simulink model "TASK1_rotating"  (R2022b)
settings: Solver=VariableStepAuto  StartTime=0.0  StopTime=3  RelTol=1e-3
values from neighbouring files (symbols this model uses):
  m = 12    [MPC_Controller.m]    (also in QP_Controller.m; TASK1_rotating_mpc.m; TASK1_walking_backward_mpc.m; TASK1_walking_forward_mpc.m)
  N = 10    [MPC_Controller.m]
undefined symbols (not defined in the file or in its folder): TASK1_rotating_mpc, X, Y, Z
libraries: sm_lib x188, nesl_utility x122, simulink x1
(part 1 of 6)
settings Model: Creator=gabemaymon  LastModifiedBy=brendanmorrison
settings ModelReferenceCC: EnableRefExpFcnMdlSchedulingChecks=on

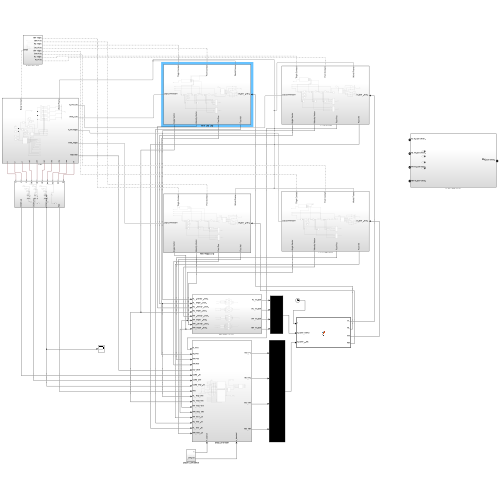
[thumbnail: Simulink's stored preview of the top-level diagram]
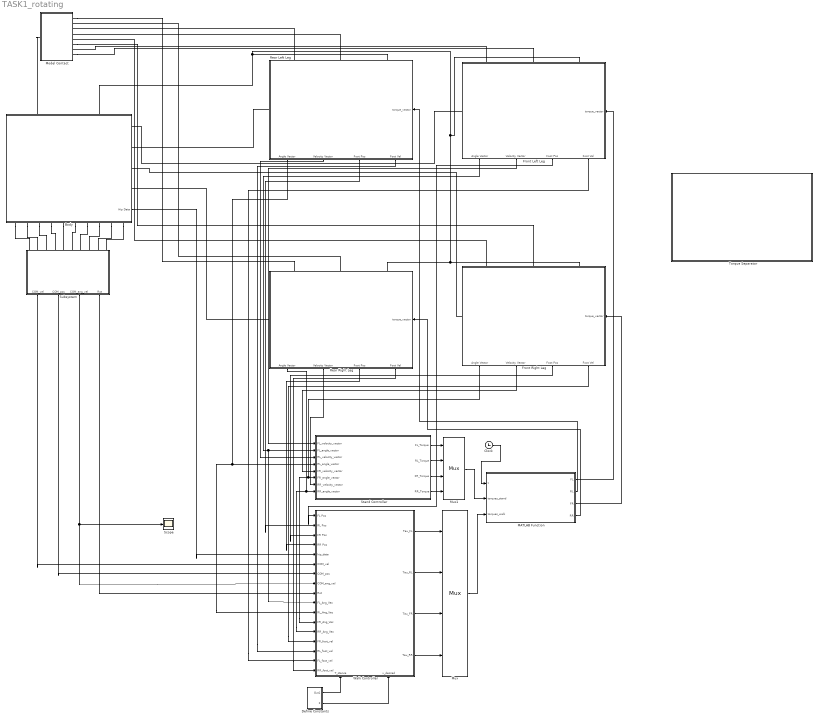
== system TASK1_rotating ==
  Body : Subsystem
      settings: PortSchema="{\"entries\":[{\"content\":{\"sides\":[{\"content\":{\"connectorIds\":[]},\"type\":\"ConnectorPlacement.EquallySpacedRectSide\",\"uuid\":\"3a53cbab-bcad-44fb-8467-9fb9b9a86323\"},{\"content\":{\"connectorIds\":[\"RConn1\",\"RConn2\",\"RConn3\",\"RConn4\",\"Out1\"],\"side\":\"RIGHT\"},\"type\":\"ConnectorPlacement.EquallySpacedRectSide\",\"uuid\":\"37b4c9a2-a58b-45a3-99d3-aa4f692e4db6\"},{\"content\":{\"connectorIds\":[\"LConn1\",\"LConn2\"],\"side\":\"TOP\"},\"type\":\"ConnectorPlacement.EquallySpacedRectSide\",\"uuid\":\"5dbc175b-de34-48ce-a2f5-f786354f8d9f\"},{\"content\":{\"connectorIds\":[\"RConn5\",\"RConn6\",\"RConn7\",\"RConn8\",\"RConn9\",\"RConn10\",\"RConn11\",\"RConn12\",\"RConn13\",\"RConn14\"],\"side\":\"BOTTOM\"},\"type\":\"ConnectorPlacement.EquallySpacedRectSide\",\"uuid\":\"77deabef-97a2-4647-8aef-301d0256e7d8\"}]},\"type\":\"ConnectorPlacement.EquallySpacedConnector\",\"uuid\":\"c3f44b19-9cb7-4370-b97a-4164cc5cfb48\"}],\"packageUris\":[\"http://schema.mathworks.com/mf0/Connector/R2020b\"],\"version\":\"1.0\"}"
  Clock : Clock
  Define Constants : Subsystem
  Front Left Leg : Subsystem
      settings: PortSchema="{\"entries\":[{\"content\":{\"sides\":[{\"content\":{\"connectorIds\":[\"LConn1\"]},\"type\":\"ConnectorPlacement.EquallySpacedRectSide\",\"uuid\":\"58990e36-5185-4bfb-924f-3ea489e575b7\"},{\"content\":{\"connectorIds\":[\"In1\"],\"side\":\"RIGHT\"},\"type\":\"ConnectorPlacement.EquallySpacedRectSide\",\"uuid\":\"00c4eac4-622f-4601-a916-f460578a2921\"},{\"content\":{\"connectorIds\":[\"LConn2\",\"LConn3\",\"LConn4\"],\"side\":\"TOP\"},\"type\":\"ConnectorPlacement.EquallySpacedRectSide\",\"uuid\":\"312df89b-6b71-4241-907b-a86e47405529\"},{\"content\":{\"connectorIds\":[\"Out1\",\"Out2\",\"Out3\",\"Out4\"],\"side\":\"BOTTOM\"},\"type\":\"ConnectorPlacement.EquallySpacedRectSide\",\"uuid\":\"0aae8fe1-113f-457b-a27e-e9cd9e6560df\"}]},\"type\":\"ConnectorPlacement.EquallySpacedConnector\",\"uuid\":\"0675262f-03c2-4ace-8aed-4bc959055a73\"}],\"packageUris\":[\"http://schema.mathworks.com/mf0/Connector/R2020b\"],\"version\":\"1.0\"}"
  Front Right Leg : Subsystem
      settings: PortSchema="{\"entries\":[{\"content\":{\"sides\":[{\"content\":{\"connectorIds\":[\"LConn1\"]},\"type\":\"ConnectorPlacement.EquallySpacedRectSide\",\"uuid\":\"58990e36-5185-4bfb-924f-3ea489e575b7\"},{\"content\":{\"connectorIds\":[\"In1\"],\"side\":\"RIGHT\"},\"type\":\"ConnectorPlacement.EquallySpacedRectSide\",\"uuid\":\"00c4eac4-622f-4601-a916-f460578a2921\"},{\"content\":{\"connectorIds\":[\"LConn2\",\"LConn3\",\"LConn4\"],\"side\":\"TOP\"},\"type\":\"ConnectorPlacement.EquallySpacedRectSide\",\"uuid\":\"312df89b-6b71-4241-907b-a86e47405529\"},{\"content\":{\"connectorIds\":[\"Out1\",\"Out2\",\"Out3\",\"Out4\"],\"side\":\"BOTTOM\"},\"type\":\"ConnectorPlacement.EquallySpacedRectSide\",\"uuid\":\"d64aa42d-2533-4acc-8ebf-5037fee0448f\"}]},\"type\":\"ConnectorPlacement.EquallySpacedConnector\",\"uuid\":\"0675262f-03c2-4ace-8aed-4bc959055a73\"}],\"packageUris\":[\"http://schema.mathworks.com/mf0/Connector/R2020b\"],\"version\":\"1.0\"}"
  MATLAB Function : MATLAB Function  TreatAsAtomicUnit=on
  Model Contact : Subsystem
  Mux : Mux
  Mux1 : Mux
  Rear Left Leg : Subsystem
      settings: PortSchema="{\"entries\":[{\"content\":{\"sides\":[{\"content\":{\"connectorIds\":[\"LConn1\"]},\"type\":\"ConnectorPlacement.EquallySpacedRectSide\",\"uuid\":\"58990e36-5185-4bfb-924f-3ea489e575b7\"},{\"content\":{\"connectorIds\":[\"In1\"],\"side\":\"RIGHT\"},\"type\":\"ConnectorPlacement.EquallySpacedRectSide\",\"uuid\":\"00c4eac4-622f-4601-a916-f460578a2921\"},{\"content\":{\"connectorIds\":[\"LConn2\",\"LConn3\",\"LConn4\"],\"side\":\"TOP\"},\"type\":\"ConnectorPlacement.EquallySpacedRectSide\",\"uuid\":\"312df89b-6b71-4241-907b-a86e47405529\"},{\"content\":{\"connectorIds\":[\"Out1\",\"Out2\",\"Out3\",\"Out4\"],\"side\":\"BOTTOM\"},\"type\":\"ConnectorPlacement.EquallySpacedRectSide\",\"uuid\":\"ff870af0-d312-4050-99ba-9f73bd605133\"}]},\"type\":\"ConnectorPlacement.EquallySpacedConnector\",\"uuid\":\"0675262f-03c2-4ace-8aed-4bc959055a73\"}],\"packageUris\":[\"http://schema.mathworks.com/mf0/Connector/R2020b\"],\"version\":\"1.0\"}"
  Rear Right Leg : Subsystem
      settings: PortSchema="{\"entries\":[{\"content\":{\"sides\":[{\"content\":{\"connectorIds\":[\"LConn1\"]},\"type\":\"ConnectorPlacement.EquallySpacedRectSide\",\"uuid\":\"58990e36-5185-4bfb-924f-3ea489e575b7\"},{\"content\":{\"connectorIds\":[\"In1\"],\"side\":\"RIGHT\"},\"type\":\"ConnectorPlacement.EquallySpacedRectSide\",\"uuid\":\"00c4eac4-622f-4601-a916-f460578a2921\"},{\"content\":{\"connectorIds\":[\"LConn2\",\"LConn3\",\"LConn4\"],\"side\":\"TOP\"},\"type\":\"ConnectorPlacement.EquallySpacedRectSide\",\"uuid\":\"312df89b-6b71-4241-907b-a86e47405529\"},{\"content\":{\"connectorIds\":[\"Out1\",\"Out2\",\"Out3\",\"Out4\"],\"side\":\"BOTTOM\"},\"type\":\"ConnectorPlacement.EquallySpacedRectSide\",\"uuid\":\"f067581c-0bad-4e2f-b908-6a87aedcf8c1\"}]},\"type\":\"ConnectorPlacement.EquallySpacedConnector\",\"uuid\":\"0675262f-03c2-4ace-8aed-4bc959055a73\"}],\"packageUris\":[\"http://schema.mathworks.com/mf0/Connector/R2020b\"],\"version\":\"1.0\"}"
  Scope : Scope
  Stand Controller : Subsystem
  Subsystem : Subsystem
  Torque Separator : Subsystem
  Walk Controller : Subsystem
      settings: PortSchema="{\"entries\":[{\"content\":{\"sides\":[{\"content\":{\"connectorIds\":[\"In1\",\"In2\",\"In3\",\"In4\",\"In5\",\"In6\",\"In7\",\"In8\",\"In9\",\"In10\",\"In11\",\"In12\",\"In13\",\"In14\",\"In15\",\"In16\",\"In17\"]},\"type\":\"ConnectorPlacement.EquallySpacedRectSide\",\"uuid\":\"1e069285-b883-4306-9ce3-c9505cac6642\"},{\"content\":{\"connectorIds\":[\"Out1\",\"Out2\",\"Out3\",\"Out4\"],\"side\":\"RIGHT\"},\"type\":\"ConnectorPlacement.EquallySpacedRectSide\",\"uuid\":\"beeabf05-15da-47f0-a05e-e3bbb85a150c\"},{\"content\":{\"connectorIds\":[],\"side\":\"TOP\"},\"type\":\"ConnectorPlacement.EquallySpacedRectSide\",\"uuid\":\"4dc75ef0-3dc8-45e4-9a6b-759a39a8569b\"},{\"content\":{\"connectorIds\":[\"In18\",\"In19\"],\"side\":\"BOTTOM\"},\"type\":\"ConnectorPlacement.EquallySpacedRectSide\",\"uuid\":\"16e05f6d-d9c2-431a-98da-de6aa17a42c7\"}]},\"type\":\"ConnectorPlacement.EquallySpacedConnector\",\"uuid\":\"7eb70f55-b335-4fe2-939a-f221a9bcbcbb\"}],\"packageUris\":[\"http://schema.mathworks.com/mf0/Connector/R2020b\"],\"version\":\"1.0\"}"
  wires:
  Front Left Leg/2(Velocity Vector) -> Stand Controller/1(FL_velocity_vector)
  Front Left Leg/1(Angle Vector) -> Walk Controller/10(FL_Ang_Vec), Stand Controller/2(FL_angle_vector)
  Rear Left Leg/1(Angle Vector) -> Walk Controller/11(RL_Ang_Vec), Stand Controller/4(RL_angle_vector)
  Rear Left Leg/2(Velocity Vector) -> Stand Controller/3(RL_velocity_vector)
  Rear Right Leg/1(Angle Vector) -> Walk Controller/13(RR_Ang_Vec), Stand Controller/8(RR_angle_vector)
  Rear Right Leg/2(Velocity Vector) -> Stand Controller/7(RR_velocity_vector)
  Front Right Leg/1(Angle Vector) -> Walk Controller/12(FR_Ang_Vec), Stand Controller/6(FR_angle_vector)
  Front Right Leg/2(Velocity Vector) -> Stand Controller/5(FR_velocity_vector)
  Stand Controller/1(FL_Torque) -> Mux1/1
  Stand Controller/2(RL_Torque) -> Mux1/2
  Stand Controller/3(FR_Torque) -> Mux1/3
  Stand Controller/4(RR_Torque) -> Mux1/4
  Mux1/1 -> MATLAB Function/2(torques_stand)
  Mux/1 -> MATLAB Function/3(torques_walk)
  MATLAB Function/1(FL) -> Front Left Leg/1(torque_vector)
  MATLAB Function/3(FR) -> Front Right Leg/1(torque_vector)
  MATLAB Function/2(RL) -> Rear Left Leg/1(torque_vector)
  MATLAB Function/4(RR) -> Rear Right Leg/1(torque_vector)
  Front Left Leg/3(" Foot Pos") -> Walk Controller/1(FL Pos)
  Rear Left Leg/3(" Foot Pos") -> Walk Controller/2(RL Pos)
  Body/1(Hip Data) -> Walk Controller/5(hip_data)
  Subsystem/1(COM_vel) -> Walk Controller/6(COM_vel)
  Subsystem/2(COM_pos) -> Walk Controller/7(COM_pos)
  Subsystem/3(COM_ang_vel) -> Walk Controller/8(COM_ang_vel), Scope/1
  Subsystem/4(Rot) -> Walk Controller/9(Rot)
  Front Right Leg/3(" Foot Pos") -> Walk Controller/3(FR Pos)
  Rear Right Leg/3(" Foot Pos") -> Walk Controller/4(RR Pos)
  Define Constants/1(Out1) -> Walk Controller/18(T_stance)
  Define Constants/2(v_desired) -> Walk Controller/19(v_desired)
  Walk Controller/1(Tau_FL) -> Mux/1
  Walk Controller/2(Tau_RL) -> Mux/2
  Walk Controller/3(Tau_FR) -> Mux/3
  Walk Controller/4(Tau_RR) -> Mux/4
  Rear Left Leg/4(" Foot Vel") -> Walk Controller/15(RL_foot_vel)
  Rear Right Leg/4(" Foot Vel") -> Walk Controller/17(RR_foot_vel)
  Front Right Leg/4(" Foot Vel") -> Walk Controller/14(FR_foot_vel)
  Front Left Leg/4(" Foot Vel") -> Walk Controller/16(FL_foot_vel)
  Clock/1 -> MATLAB Function/1(t)
  connections:
  Model Contact/RConn1 -- Rear Right Leg/LConn2
  Rear Left Leg/LConn2 -- Model Contact/RConn3
  Front Right Leg/LConn2 -- Model Contact/RConn5
  Front Left Leg/LConn2 -- Model Contact/RConn7
  Rear Right Leg/LConn3 -- Model Contact/RConn2
  Rear Left Leg/LConn3 -- Model Contact/RConn4
  Model Contact/RConn6 -- Front Right Leg/LConn3
  Model Contact/RConn8 -- Front Left Leg/LConn3
  Model Contact/LConn1 -- Body/LConn1
  Front Right Leg/LConn1 -- Body/RConn3
  Rear Left Leg/LConn1 -- Body/RConn2
  Rear Right Leg/LConn1 -- Body/RConn4
  Front Left Leg/LConn1 -- Body/RConn1
  Body/LConn2 -- Front Left Leg/LConn4 -- Front Right Leg/LConn4 -- Rear Right Leg/LConn4 -- Rear Left Leg/LConn4
  Body/RConn5 -- Subsystem/LConn1
  Body/RConn6 -- Subsystem/LConn2
  Body/RConn7 -- Subsystem/LConn3
  Body/RConn8 -- Subsystem/LConn4
  Body/RConn9 -- Subsystem/LConn5
  Body/RConn10 -- Subsystem/LConn6
  Body/RConn11 -- Subsystem/LConn7
  Body/RConn12 -- Subsystem/LConn8
  Body/RConn13 -- Subsystem/LConn9
  Body/RConn14 -- Subsystem/LConn10

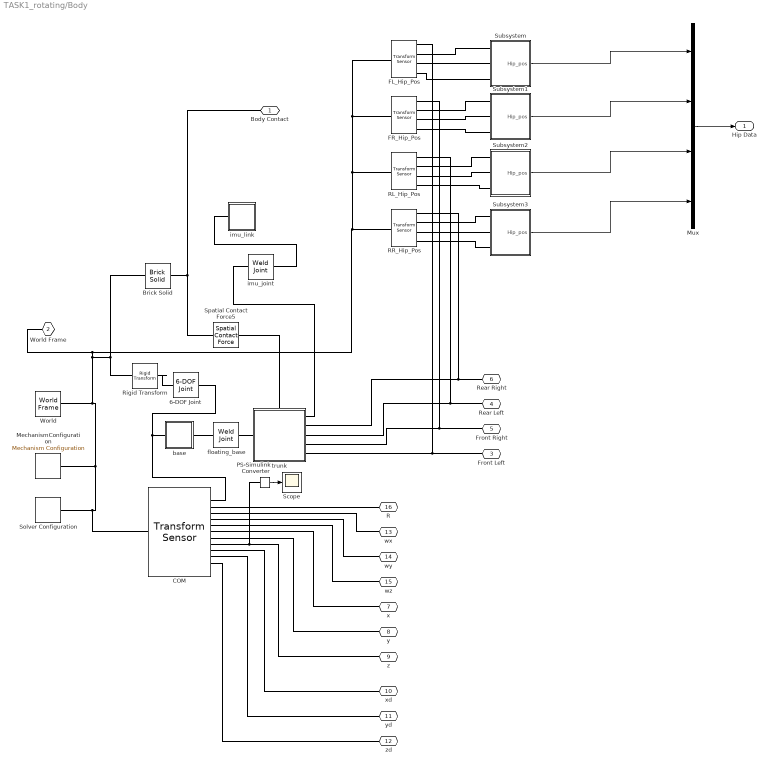
== system TASK1_rotating/Body ==
  " COM" : sm_lib/Frames and Transforms/Transform Sensor  MeasurementFrame=World  SenseAngle=off  SenseAxis=off  SenseQ=off  SenseR=on  SenseRotationSequence=off  RotationSequence=XYX  SenseOmegaX=on  SenseOmegaY=on  SenseOmegaZ=on  SenseQDot=off  SenseRDot=off  SenseAlphaX=off  SenseAlphaY=off  SenseAlphaZ=off  SenseQDDot=off  SenseRDDot=off  SenseX=on  SenseY=on  SenseZ=on  SenseRad=off  SenseAzim=off  SenseDist=off  SenseInc=off  SenseXDot=on  SenseYDot=on  SenseZDot=on  SenseRadDot=off  SenseAzimDot=off  SenseDistDot=off  SenseIncDot=off  SenseXDDot=off  SenseYDDot=off  SenseZDDot=off  SenseRadDDot=off  SenseAzimDDot=off  SenseDistDDot=off  SenseIncDDot=off
  6-DOF Joint : sm_lib/Joints/6-DOF Joint  JointMode=Normal  SenseConstraintForce=off  SenseConstraintForceX=off  SenseConstraintForceY=off  SenseConstraintForceZ=off  SenseConstraintTorque=off  SenseConstraintTorqueX=off  SenseConstraintTorqueY=off  SenseConstraintTorqueZ=off  SenseTotalForce=off  SenseTotalForceX=off  SenseTotalForceY=off  SenseTotalForceZ=off  SenseTotalTorque=off  SenseTotalTorqueX=off  SenseTotalTorqueY=off  SenseTotalTorqueZ=off  CompositeWrenchDir=FollowerOnBase  CompositeWrenchFrame=BaseFrame  PxEquilibriumPosition=0  PxEquilibriumPositionUnits=m  PxSpringStiffness=0  PxSpringStiffnessUnits=N/m  PxDampingCoefficient=0  PxDampingCoefficientUnits=N/(m/s)  PxTorqueActuationMode=NoTorque  PxMotionActuationMode=ComputedMotion  PxSensePosition=off  PxSenseVelocity=off  PxSenseAcceleration=off  PxSenseTorqueForce=off  PxSenseLowerLimitTorqueForce=off  PxSenseUpperLimitTorqueForce=off  PxLowerLimitSpecify=off  PxLowerLimitBound=-1  PxLowerLimitBoundUnits=m  PxLowerLimitStiffness=1e6  PxLowerLimitStiffnessUnits=N/m  PxLowerLimitDamping=1e3  PxLowerLimitDampingUnits=N/(m/s)  PxLowerLimitTransitionRegionWidth=1e-4  PxLowerLimitTransitionRegionWidthUnits=m  PxUpperLimitSpecify=off  PxUpperLimitBound=1  PxUpperLimitBoundUnits=m  PxUpperLimitStiffness=1e6  PxUpperLimitStiffnessUnits=N/m  PxUpperLimitDamping=1e3  PxUpperLimitDampingUnits=N/(m/s)  PxUpperLimitTransitionRegionWidth=1e-4  PxUpperLimitTransitionRegionWidthUnits=m  PxPositionTargetSpecify=off  PxPositionTargetPriority=High  PxPositionTargetValue=0  PxPositionTargetValueUnits=m  PxVelocityTargetSpecify=off  PxVelocityTargetPriority=High  PxVelocityTargetValue=0  PxVelocityTargetValueUnits=m/s  PyEquilibriumPosition=0  PyEquilibriumPositionUnits=m  PySpringStiffness=0  PySpringStiffnessUnits=N/m  PyDampingCoefficient=0  PyDampingCoefficientUnits=N/(m/s)  PyTorqueActuationMode=NoTorque  PyMotionActuationMode=ComputedMotion  PySensePosition=off  PySenseVelocity=off  PySenseAcceleration=off  PySenseTorqueForce=off  PySenseLowerLimitTorqueForce=off  PySenseUpperLimitTorqueForce=off  PyLowerLimitSpecify=off  PyLowerLimitBound=-1  PyLowerLimitBoundUnits=m  PyLowerLimitStiffness=1e6  PyLowerLimitStiffnessUnits=N/m  PyLowerLimitDamping=1e3  PyLowerLimitDampingUnits=N/(m/s)  PyLowerLimitTransitionRegionWidth=1e-4  PyLowerLimitTransitionRegionWidthUnits=m  PyUpperLimitSpecify=off  PyUpperLimitBound=1  PyUpperLimitBoundUnits=m  PyUpperLimitStiffness=1e6  PyUpperLimitStiffnessUnits=N/m  PyUpperLimitDamping=1e3  PyUpperLimitDampingUnits=N/(m/s)  PyUpperLimitTransitionRegionWidth=1e-4  PyUpperLimitTransitionRegionWidthUnits=m  PyPositionTargetSpecify=off  PyPositionTargetPriority=High  PyPositionTargetValue=0  PyPositionTargetValueUnits=m  PyVelocityTargetSpecify=off  PyVelocityTargetPriority=High  PyVelocityTargetValue=0  PyVelocityTargetValueUnits=m/s  PzEquilibriumPosition=0  PzEquilibriumPositionUnits=m  PzSpringStiffness=0  PzSpringStiffnessUnits=N/m  PzDampingCoefficient=0  PzDampingCoefficientUnits=N/(m/s)  PzTorqueActuationMode=NoTorque  PzMotionActuationMode=ComputedMotion  PzSensePosition=off  PzSenseVelocity=off  PzSenseAcceleration=off  PzSenseTorqueForce=off  PzSenseLowerLimitTorqueForce=off  PzSenseUpperLimitTorqueForce=off  PzLowerLimitSpecify=off  PzLowerLimitBound=-1  PzLowerLimitBoundUnits=m  PzLowerLimitStiffness=1e6  PzLowerLimitStiffnessUnits=N/m  PzLowerLimitDamping=1e3  PzLowerLimitDampingUnits=N/(m/s)  PzLowerLimitTransitionRegionWidth=1e-4  PzLowerLimitTransitionRegionWidthUnits=m  PzUpperLimitSpecify=off  PzUpperLimitBound=1  PzUpperLimitBoundUnits=m  PzUpperLimitStiffness=1e6  PzUpperLimitStiffnessUnits=N/m  PzUpperLimitDamping=1e3  PzUpperLimitDampingUnits=N/(m/s)  PzUpperLimitTransitionRegionWidth=1e-4  PzUpperLimitTransitionRegionWidthUnits=m  PzPositionTargetSpecify=off  PzPositionTargetPriority=High  PzPositionTargetValue=0  PzPositionTargetValueUnits=m  PzVelocityTargetSpecify=off  PzVelocityTargetPriority=High  PzVelocityTargetValue=0  PzVelocityTargetValueUnits=m/s  SphEqPosRotationMethod=None  SphEqPosRotationAngleUnits=deg  SphEqPosRotationStandardAxis=+Z  SphEqPosRotationAngle=0.0  SphEqPosRotationArbitraryAxis=[0 0 1]  SphEqPosFollAlignAxisA=+X  SphEqPosBaseAlignAxisA=+Y  SphEqPosFollAlignAxisB=+Y  SphEqPosBaseAlignAxisB=+Z  SphEqPosRotationSequenceAxes=FollowerAxes  SphEqPosRotationSequence=XYX  SphEqPosRotationSequenceAngles=[0 0 0]  SphEqPosRotationSequenceAnglesUnits=deg  SphEqPosRotationMatrix=[1 0 0; 0 1 0; 0 0 1]  SphEqPosQuaternion=[1 0 0 0]  SphSpringStiffness=0  SphSpringStiffnessUnits=N*m/deg  SphDampingCoefficient=0  SphDampingCoefficientUnits=N*m/(deg/s)  SphActuateTorqueX=off  SphActuateTorqueY=off  SphActuateTorqueZ=off  SphActuateTorque=off  SphTorqueActuationMode=NoTorque  SphMotionActuationMode=ComputedMotion  SphActuationFrame=BaseFrame  SphSensePosition=off  SphSenseVelocityX=off  SphSenseVelocityY=off  SphSenseVelocityZ=off  SphSenseVelocity=off  SphSenseAccelerationX=off  SphSenseAccelerationY=off  SphSenseAccelerationZ=off  SphSenseAcceleration=off  SphSenseTorqueX=off  SphSenseTorqueY=off  SphSenseTorqueZ=off  SphSenseTorqueForce=off  SphSenseLowerLimitTorqueMag=off  SphSenseUpperLimitTorqueMag=off  SphSensingFrame=BaseFrame  SphLowerLimitSpecify=off  SphLowerLimitBound=15  SphLowerLimitBoundUnits=deg  SphLowerLimitStiffness=1e4  SphLowerLimitStiffnessUnits=N*m/deg  SphLowerLimitDamping=10  SphLowerLimitDampingUnits=N*m/(deg/s)  SphLowerLimitTransitionRegionWidth=0.1  SphLowerLimitTransitionRegionWidthUnits=deg  SphUpperLimitSpecify=off  SphUpperLimitBound=45  SphUpperLimitBoundUnits=deg  SphUpperLimitStiffness=1e4  SphUpperLimitStiffnessUnits=N*m/deg  SphUpperLimitDamping=10  SphUpperLimitDampingUnits=N*m/(deg/s)  SphUpperLimitTransitionRegionWidth=0.1  SphUpperLimitTransitionRegionWidthUnits=deg  SphPositionTargetRotationMethod=None  SphPositionTargetRotationAngleUnits=deg  SphPositionTargetRotationStandardAxis=+Z  SphPositionTargetRotationAngle=0.0  SphPositionTargetRotationArbitraryAxis=[0 0 1]  SphPositionTargetFollAlignAxisA=+X  SphPositionTargetBaseAlignAxisA=+Y  SphPositionTargetFollAlignAxisB=+Y  SphPositionTargetBaseAlignAxisB=+Z  SphPositionTargetRotationSequenceAxes=FollowerAxes  SphPositionTargetRotationSequence=XYX  SphPositionTargetRotationSequenceAngles=[0 0 0]  SphPositionTargetRotationSequenceAnglesUnits=deg  SphPositionTargetRotationMatrix=[1 0 0; 0 1 0; 0 0 1]  SphPositionTargetQuaternion=[1 0 0 0]  SphPositionTargetSpecify=off  SphPositionTargetPriority=High  SphVelocityTargetValue=[0 0 0]  SphVelocityTargetValueUnits=deg/s  SphVelocityTargetSpecify=off  SphVelocityTargetPriority=High  SphVelocityTargetInFollowerFrame=on
  Brick Solid : sm_lib/Body Elements/Brick Solid  GraphicAmbientColor=[0.15 0.15 0.15 1.0]  BasedOnType=Density  BrickDimensions=[3 3 0.01]  BrickDimensionUnits=m  CenterOfMass=[0 0 0]  CenterOfMassUnits=m  GraphicDiffuseColor=[0.5 0.5 0.5]  Density=1000  DensityUnits=kg/m^3  DoExposeReferenceFrame=off  GraphicEmissiveColor=[0.0 0.0 0.0 1.0]  ExportEntireGeometry=on  SerializedFrames=<Frames><Frame><Id>Frame1</Id><Value><Name>F1</Name><Origin><Source>GeometricFeature</Source><FeatureName>+z surface</FeatureName></Origin><PrimaryAxis><DefinedDirection>+Z</DefinedDirection><Source>ReferenceFrame</Source><SourceDirection>+Z</SourceDirection><FeatureName></FeatureName></PrimaryAxis><SecondaryAxis><DefinedDirection>+X</DefinedDirection><Source>ReferenceFrame</Source><SourceDirection>+X</SourceDirection><FeatureName></FeatureName></SecondaryAxis></Value></Frame></Frames>  MarkerShape=Sphere  MarkerSize=10  GraphicType=FromGeometry  InertiaType=CalculateFromGeometry  Mass=1  MassUnits=kg  MomentsOfInertia=[1 1 1]  MomentsOfInertiaUnits=kg*m^2  GraphicOpacity=1.0  ProductsOfInertia=[0 0 0]  ProductsOfInertiaUnits=kg*m^2  GraphicShininess=75  GraphicSpecularColor=[0.5 0.5 0.5 1.0]  GraphicVisPropType=SimpleVisualProperties
  FL_Hip_Pos : sm_lib/Frames and Transforms/Transform Sensor  MeasurementFrame=World  SenseAngle=off  SenseAxis=off  SenseQ=off  SenseR=off  SenseRotationSequence=off  RotationSequence=XYX  SenseOmegaX=off  SenseOmegaY=off  SenseOmegaZ=off  SenseQDot=off  SenseRDot=off  SenseAlphaX=off  SenseAlphaY=off  SenseAlphaZ=off  SenseQDDot=off  SenseRDDot=off  SenseX=on  SenseY=on  SenseZ=on  SenseRad=off  SenseAzim=off  SenseDist=off  SenseInc=off  SenseXDot=off  SenseYDot=off  SenseZDot=off  SenseRadDot=off  SenseAzimDot=off  SenseDistDot=off  SenseIncDot=off  SenseXDDot=off  SenseYDDot=off  SenseZDDot=off  SenseRadDDot=off  SenseAzimDDot=off  SenseDistDDot=off  SenseIncDDot=off
  FR_Hip_Pos : sm_lib/Frames and Transforms/Transform Sensor  MeasurementFrame=World  SenseAngle=off  SenseAxis=off  SenseQ=off  SenseR=off  SenseRotationSequence=off  RotationSequence=XYX  SenseOmegaX=off  SenseOmegaY=off  SenseOmegaZ=off  SenseQDot=off  SenseRDot=off  SenseAlphaX=off  SenseAlphaY=off  SenseAlphaZ=off  SenseQDDot=off  SenseRDDot=off  SenseX=on  SenseY=on  SenseZ=on  SenseRad=off  SenseAzim=off  SenseDist=off  SenseInc=off  SenseXDot=off  SenseYDot=off  SenseZDot=off  SenseRadDot=off  SenseAzimDot=off  SenseDistDot=off  SenseIncDot=off  SenseXDDot=off  SenseYDDot=off  SenseZDDot=off  SenseRadDDot=off  SenseAzimDDot=off  SenseDistDDot=off  SenseIncDDot=off
  MechanismConfiguration : sm_lib/Utilities/Mechanism Configuration  UniformGravity=Constant  GravityVector=[0 0 -9.8]  GravityUnits=m/s^2  LinearizationDelta=0.001  JointModeTransitionNonlinearIterations=2
  Mux : Mux
  PS-Simulink Converter : nesl_utility/PS-Simulink Converter  PhysicalDomain=network_engine_domain  SubClassName=ps_output  LeftPortType=input  RightPortType=output  PseudoPeriodic=off  Frequencies=[]  VectorFormat=inherit  Unit=inherit  AffineConversion=off
  RL_Hip_Pos : sm_lib/Frames and Transforms/Transform Sensor  MeasurementFrame=World  SenseAngle=off  SenseAxis=off  SenseQ=off  SenseR=off  SenseRotationSequence=off  RotationSequence=XYX  SenseOmegaX=off  SenseOmegaY=off  SenseOmegaZ=off  SenseQDot=off  SenseRDot=off  SenseAlphaX=off  SenseAlphaY=off  SenseAlphaZ=off  SenseQDDot=off  SenseRDDot=off  SenseX=on  SenseY=on  SenseZ=on  SenseRad=off  SenseAzim=off  SenseDist=off  SenseInc=off  SenseXDot=off  SenseYDot=off  SenseZDot=off  SenseRadDot=off  SenseAzimDot=off  SenseDistDot=off  SenseIncDot=off  SenseXDDot=off  SenseYDDot=off  SenseZDDot=off  SenseRadDDot=off  SenseAzimDDot=off  SenseDistDDot=off  SenseIncDDot=off
  RR_Hip_Pos : sm_lib/Frames and Transforms/Transform Sensor  MeasurementFrame=World  SenseAngle=off  SenseAxis=off  SenseQ=off  SenseR=off  SenseRotationSequence=off  RotationSequence=XYX  SenseOmegaX=off  SenseOmegaY=off  SenseOmegaZ=off  SenseQDot=off  SenseRDot=off  SenseAlphaX=off  SenseAlphaY=off  SenseAlphaZ=off  SenseQDDot=off  SenseRDDot=off  SenseX=on  SenseY=on  SenseZ=on  SenseRad=off  SenseAzim=off  SenseDist=off  SenseInc=off  SenseXDot=off  SenseYDot=off  SenseZDot=off  SenseRadDot=off  SenseAzimDot=off  SenseDistDot=off  SenseIncDot=off  SenseXDDot=off  SenseYDDot=off  SenseZDDot=off  SenseRadDDot=off  SenseAzimDDot=off  SenseDistDDot=off  SenseIncDDot=off
  Rigid Transform : sm_lib/Frames and Transforms/Rigid Transform  TranslationMethod=Cartesian  TranslationStandardOffset=0  TranslationLengthUnit=m  TranslationStandardAxis=+Z  TranslationCartesianOffset=[0 0 0.13]  TranslationROffset=0  TranslationROffsetUnits=m  TranslationZOffset=0  TranslationZOffsetUnits=m  TranslationThetaOffset=0  TranslationThetaOffsetUnits=deg  RotationMethod=StandardAxis  RotationAngleUnits=rad  RotationStandardAxis=+Z  RotationAngle=0  RotationArbitraryAxis=[0 0 1]  FollAlignAxisA=+X  BaseAlignAxisA=+Y  FollAlignAxisB=+Y  BaseAlignAxisB=+Z  RotationSequenceAxes=FollowerAxes  RotationSequence=XYX  RotationSequenceAngles=[0 0 0]  RotationSequenceAnglesUnits=deg  RotationMatrix=[1 0 0; 0 1 0; 0 0 1]  Quaternion=[1 0 0 0]
  Scope : Scope
  Solver Configuration : nesl_utility/Solver Configuration  PhysicalDomain=network_engine_domain  SubClassName=solver  LeftPortType=input  RightPortType=generic  Tones=[]  Harmonics=[]  SimulateNoise=off  Profile=off  UseLocalSampling=off  EnableSwitchedLinearOptims=on  FrequencyDomain=off  UseCCode=off  RelTol=0.001  AbsTol=0.001  MinStep=1e-09  ToWorkspace=off  RevertToSquareIcSolve=off  NumHomotopyIterations=100  PhasorMode=off  PhasorModeNumHarmonics=1  ConsistencySolver=NEWTON_FTOL  IndexReductionMethod=DerivativeReplacement  DoDC=off  ResidualTolerance=1e-09  ConsistencyTolSource=GLOBAL  ConsistencyAbsTol=0.001  ConsistencyRelTol=0.001  ConsistencyTolFactor=0.001  UseLocalSolver=off  LocalSolverChoice=NE_BACKWARD_EULER_ADVANCER  ResolveIndetEquations=on  FunctionEvalNumThread=1  LocalSolverSampleTime=0.001  DoFixedCost=off  MaxNonlinIter=3  MaxModeIter=2  ComputeImpulses=off  ImpulseIterations=2  LinearAlgebra=auto  LinearAlgebraNumThread=0  EquationFormulation=NE_TIME_EF  DelaysMemoryBudget=1024  AutomaticFiltering=on  FilteringTimeConstant=0.001  PartitionStorageMethod=AS_NEEDED  PartitionMemoryBudget=1024  PartitionMethod=ROBUST
  Spatial Contact Force5 : sm_lib/Forces and Torques/Spatial Contact Force  SenseContactBaseRotation=off  SenseContactBaseTranslation=off  CoefficientOfDynamicFriction=0.3  CoefficientOfStaticFriction=0.5  NormalDamping=1e3  NormalDampingUnits=N/(m/s)  SenseContactSignal=off  NormalStiffness=1e6  NormalStiffnessUnits=N/m  FrictionalCriticalVelocity=1e-3  FrictionalCriticalVelocityUnits=m/s  ZeroCrossDetectContactStartAndEnd=off  SenseContactFollowerRotation=off  SenseContactFollowerTranslation=off  FrictionType=SmoothStickSlip  SenseFrictionalForceMagnitude=off  SenseNormalForceMagnitude=off  NormalForceType=SmoothSpringDamper  SenseNormalVelocity=off  SenseSeparationDistance=off  SenseTangentialVelocity=off  NormalTransitionRegionWidth=1e-4  NormalTransitionRegionWidthUnits=m
  Subsystem : Subsystem
  Subsystem1 : Subsystem
  Subsystem2 : Subsystem
  Subsystem3 : Subsystem
  World : sm_lib/Frames and Transforms/World Frame
  base : Subsystem
  floating_base : sm_lib/Joints/Weld Joint  JointMode=Normal  SenseConstraintForce=off  SenseConstraintForceX=off  SenseConstraintForceY=off  SenseConstraintForceZ=off  SenseConstraintTorque=off  SenseConstraintTorqueX=off  SenseConstraintTorqueY=off  SenseConstraintTorqueZ=off  SenseTotalForce=off  SenseTotalForceX=off  SenseTotalForceY=off  SenseTotalForceZ=off  SenseTotalTorque=off  SenseTotalTorqueX=off  SenseTotalTorqueY=off  SenseTotalTorqueZ=off  CompositeWrenchDir=FollowerOnBase  CompositeWrenchFrame=BaseFrame
  imu_joint : sm_lib/Joints/Weld Joint  JointMode=Normal  SenseConstraintForce=off  SenseConstraintForceX=off  SenseConstraintForceY=off  SenseConstraintForceZ=off  SenseConstraintTorque=off  SenseConstraintTorqueX=off  SenseConstraintTorqueY=off  SenseConstraintTorqueZ=off  SenseTotalForce=off  SenseTotalForceX=off  SenseTotalForceY=off  SenseTotalForceZ=off  SenseTotalTorque=off  SenseTotalTorqueX=off  SenseTotalTorqueY=off  SenseTotalTorqueZ=off  CompositeWrenchDir=FollowerOnBase  CompositeWrenchFrame=BaseFrame
  imu_link : Subsystem
  trunk : Subsystem
      settings: PortSchema="{\"entries\":[{\"content\":{\"sides\":[{\"content\":{\"connectorIds\":[\"LConn1\"]},\"type\":\"ConnectorPlacement.EquallySpacedRectSide\",\"uuid\":\"c5dfde28-9f4a-41b5-9a32-9d7a562ca9b8\"},{\"content\":{\"connectorIds\":[\"RConn1\",\"RConn2\",\"RConn3\",\"RConn4\",\"RConn5\"],\"side\":\"RIGHT\"},\"type\":\"ConnectorPlacement.EquallySpacedRectSide\",\"uuid\":\"181a9597-adfa-43f0-a8d0-b0dc8d73bccd\"},{\"content\":{\"connectorIds\":[\"LConn2\"],\"side\":\"TOP\"},\"type\":\"ConnectorPlacement.EquallySpacedRectSide\",\"uuid\":\"c0b6f85e-7be1-46d7-a6dd-cb433a6623c5\"}]},\"type\":\"ConnectorPlacement.EquallySpacedConnector\",\"uuid\":\"d5811d83-3447-4618-805d-5c853b175af3\"}],\"packageUris\":[\"http://schema.mathworks.com/mf0/Connector/R2020b\"],\"version\":\"1.0\"}"
  Body Contact : PMIOPort  Side=Left
  World Frame : PMIOPort  Port=2  Side=Left
  Front Left : PMIOPort  Port=3  Side=Right
  Rear Left : PMIOPort  Port=4  Side=Right
  Front Right : PMIOPort  Port=5  Side=Right
  Rear Right : PMIOPort  Port=6  Side=Right
  x : PMIOPort  Port=7  Side=Right
  y : PMIOPort  Port=8  Side=Right
  z : PMIOPort  Port=9  Side=Right
  xd : PMIOPort  Port=10  Side=Right
  yd : PMIOPort  Port=11  Side=Right
  zd : PMIOPort  Port=12  Side=Right
  wx : PMIOPort  Port=13  Side=Right
  wy : PMIOPort  Port=14  Side=Right
  wz : PMIOPort  Port=15  Side=Right
  R : PMIOPort  Port=16  Side=Right
  Hip Data : Outport
  wires:
  PS-Simulink Converter/1 -> Scope/1
  Mux/1 -> Hip Data/1
  Subsystem2/1(Hip_pos) -> Mux/3
  Subsystem1/1(Hip_pos) -> Mux/2
  Subsystem3/1(Hip_pos) -> Mux/4
  Subsystem/1(Hip_pos) -> Mux/1
  connections:
  Front Left/RConn1 -- FL_Hip_Pos/RConn1 -- trunk/RConn5
  " COM"/RConn5 -- wz/RConn1
  imu_joint/LConn1 -- trunk/RConn1
  " COM"/RConn11 -- zd/RConn1
  " COM"/RConn9 -- xd/RConn1
  " COM"/RConn7 -- y/RConn1
  " COM"/RConn2 -- R/RConn1
  " COM"/RConn10 -- yd/RConn1
  Spatial Contact Force5/RConn1 -- trunk/LConn2
  " COM"/RConn4 -- wy/RConn1
  " COM"/RConn8 -- PS-Simulink Converter/LConn1 -- z/RConn1
  imu_joint/RConn1 -- imu_link/LConn1
  Spatial Contact Force5/LConn1 -- Body Contact/RConn1 -- Brick Solid/RConn1
  Rear Left/RConn1 -- RL_Hip_Pos/RConn1 -- trunk/RConn3
  floating_base/RConn1 -- trunk/LConn1
  Front Right/RConn1 -- FR_Hip_Pos/RConn1 -- trunk/RConn4
  " COM"/RConn6 -- x/RConn1
  World/RConn1 -- FL_Hip_Pos/LConn1 -- FR_Hip_Pos/LConn1 -- RL_Hip_Pos/LConn1 -- RR_Hip_Pos/LConn1 -- World Frame/RConn1 -- Brick Solid/LConn1 -- Rigid Transform/LConn1 -- " COM"/LConn1 -- Solver Configuration/RConn1 -- MechanismConfiguration/RConn1
  6-DOF Joint/RConn1 -- " COM"/RConn1 -- base/LConn1
  Rigid Transform/RConn1 -- 6-DOF Joint/LConn1
  " COM"/RConn3 -- wx/RConn1
  base/RConn1 -- floating_base/LConn1
  Rear Right/RConn1 -- RR_Hip_Pos/RConn1 -- trunk/RConn2
  Subsystem/LConn1 -- FL_Hip_Pos/RConn2
  FL_Hip_Pos/RConn3 -- Subsystem/LConn2
  FL_Hip_Pos/RConn4 -- Subsystem/LConn3
  FR_Hip_Pos/RConn2 -- Subsystem1/LConn1
  FR_Hip_Pos/RConn3 -- Subsystem1/LConn2
  FR_Hip_Pos/RConn4 -- Subsystem1/LConn3
  RL_Hip_Pos/RConn2 -- Subsystem2/LConn1
  RL_Hip_Pos/RConn3 -- Subsystem2/LConn2
  RL_Hip_Pos/RConn4 -- Subsystem2/LConn3
  RR_Hip_Pos/RConn2 -- Subsystem3/LConn1
  RR_Hip_Pos/RConn3 -- Subsystem3/LConn2
  RR_Hip_Pos/RConn4 -- Subsystem3/LConn3

== system TASK1_rotating/Define Constants ==
  Mux : Mux  Inputs=3
  Ramp : simulink/Sources/Ramp  slope=0.1  start=1  InitialOutput=0
  Saturation : Saturate
  Scope : Scope
  Switch : Switch  Criteria=u2 > Threshold  Threshold=0.5  SaturateOnIntegerOverflow=off  InputSameDT=off
  T_stance : Constant  Value=0.2
  Vx_desired : Constant  Value=0
  Vy_desired : Constant  Value=0
  Vz_desired : Constant  Value=0
  Out1 : Outport
  v_desired : Outport  Port=2
  wires:
  Mux/1 -> v_desired/1
  T_stance/1 -> Out1/1
  Vz_desired/1 -> Mux/3
  Ramp/1 -> Saturation/1
  Vx_desired/1 -> Mux/1
  Saturation/1 -> Scope/1, Mux/2

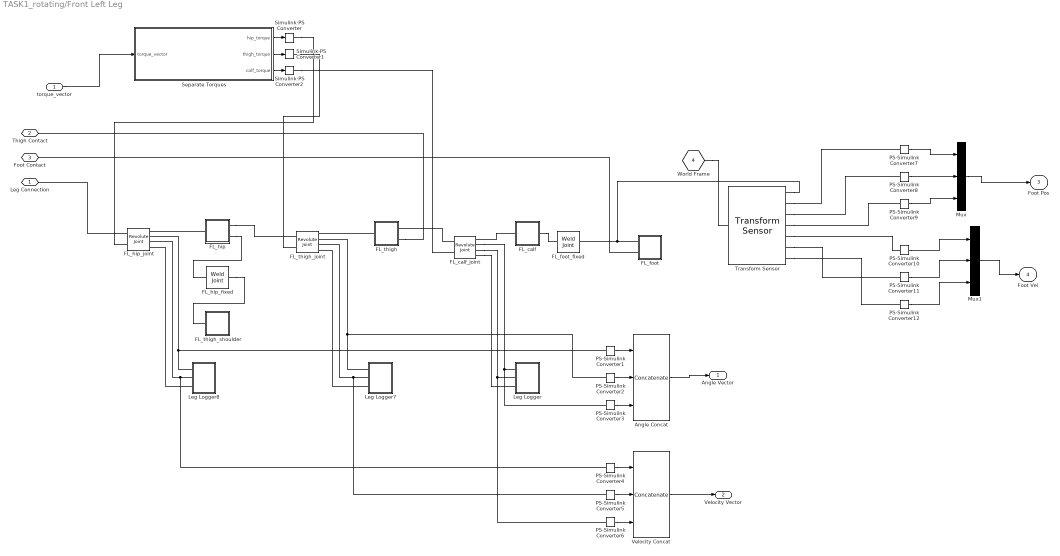
== system TASK1_rotating/Front Left Leg ==
  torque_vector : Inport
  Angle Concat : Concatenate  NumInputs=3
  FL_calf : Subsystem
  FL_calf_joint : sm_lib/Joints/Revolute Joint  JointMode=Normal  SenseConstraintForce=off  SenseConstraintForceX=off  SenseConstraintForceY=off  SenseConstraintForceZ=off  SenseConstraintTorque=off  SenseConstraintTorqueX=off  SenseConstraintTorqueY=off  SenseConstraintTorqueZ=off  SenseTotalForce=off  SenseTotalForceX=off  SenseTotalForceY=off  SenseTotalForceZ=off  SenseTotalTorque=off  SenseTotalTorqueX=off  SenseTotalTorqueY=off  SenseTotalTorqueZ=off  CompositeWrenchDir=FollowerOnBase  CompositeWrenchFrame=BaseFrame  EquilibriumPosition=0  EquilibriumPositionUnits=deg  SpringStiffness=0  SpringStiffnessUnits=N*m/deg  DampingCoefficient=0.01  DampingCoefficientUnits=kg*m^2/(rad*s)  TorqueActuationMode=InputTorque  MotionActuationMode=ComputedMotion  SensePosition=on  SenseVelocity=on  SenseAcceleration=off  SenseTorqueForce=on  SenseLowerLimitTorqueForce=off  SenseUpperLimitTorqueForce=off  LowerLimitSpecify=on  LowerLimitBound=-2.69653369433  LowerLimitBoundUnits=rad  LowerLimitStiffness=1e4  LowerLimitStiffnessUnits=N*m/deg  LowerLimitDamping=10  LowerLimitDampingUnits=N*m/(deg/s)  LowerLimitTransitionRegionWidth=0.1  LowerLimitTransitionRegionWidthUnits=deg  UpperLimitSpecify=on  UpperLimitBound=-0.916297857297  UpperLimitBoundUnits=rad  UpperLimitStiffness=1e4  UpperLimitStiffnessUnits=N*m/deg  UpperLimitDamping=10  UpperLimitDampingUnits=N*m/(deg/s)  UpperLimitTransitionRegionWidth=0.1  UpperLimitTransitionRegionWidthUnits=deg  PositionTargetSpecify=on  PositionTargetPriority=High  PositionTargetValue=-2.5  PositionTargetValueUnits=rad  VelocityTargetSpecify=on  VelocityTargetPriority=High  VelocityTargetValue=0  VelocityTargetValueUnits=rad/s
  FL_foot : Subsystem
  FL_foot_fixed : sm_lib/Joints/Weld Joint  JointMode=Normal  SenseConstraintForce=off  SenseConstraintForceX=off  SenseConstraintForceY=off  SenseConstraintForceZ=off  SenseConstraintTorque=off  SenseConstraintTorqueX=off  SenseConstraintTorqueY=off  SenseConstraintTorqueZ=off  SenseTotalForce=off  SenseTotalForceX=off  SenseTotalForceY=off  SenseTotalForceZ=off  SenseTotalTorque=off  SenseTotalTorqueX=off  SenseTotalTorqueY=off  SenseTotalTorqueZ=off  CompositeWrenchDir=FollowerOnBase  CompositeWrenchFrame=BaseFrame
  FL_hip : Subsystem
  FL_hip_fixed : sm_lib/Joints/Weld Joint  JointMode=Normal  SenseConstraintForce=off  SenseConstraintForceX=off  SenseConstraintForceY=off  SenseConstraintForceZ=off  SenseConstraintTorque=off  SenseConstraintTorqueX=off  SenseConstraintTorqueY=off  SenseConstraintTorqueZ=off  SenseTotalForce=off  SenseTotalForceX=off  SenseTotalForceY=off  SenseTotalForceZ=off  SenseTotalTorque=off  SenseTotalTorqueX=off  SenseTotalTorqueY=off  SenseTotalTorqueZ=off  CompositeWrenchDir=FollowerOnBase  CompositeWrenchFrame=BaseFrame
  FL_hip_joint : sm_lib/Joints/Revolute Joint  JointMode=Normal  SenseConstraintForce=off  SenseConstraintForceX=off  SenseConstraintForceY=off  SenseConstraintForceZ=off  SenseConstraintTorque=off  SenseConstraintTorqueX=off  SenseConstraintTorqueY=off  SenseConstraintTorqueZ=off  SenseTotalForce=off  SenseTotalForceX=off  SenseTotalForceY=off  SenseTotalForceZ=off  SenseTotalTorque=off  SenseTotalTorqueX=off  SenseTotalTorqueY=off  SenseTotalTorqueZ=off  CompositeWrenchDir=FollowerOnBase  CompositeWrenchFrame=BaseFrame  EquilibriumPosition=0  EquilibriumPositionUnits=deg  SpringStiffness=0  SpringStiffnessUnits=N*m/deg  DampingCoefficient=0.01  DampingCoefficientUnits=kg*m^2/(rad*s)  TorqueActuationMode=InputTorque  MotionActuationMode=ComputedMotion  SensePosition=on  SenseVelocity=on  SenseAcceleration=off  SenseTorqueForce=on  SenseLowerLimitTorqueForce=off  SenseUpperLimitTorqueForce=off  LowerLimitSpecify=on  LowerLimitBound=-0.802851455917  LowerLimitBoundUnits=rad  LowerLimitStiffness=1e4  LowerLimitStiffnessUnits=N*m/deg  LowerLimitDamping=10  LowerLimitDampingUnits=N*m/(deg/s)  LowerLimitTransitionRegionWidth=0.1  LowerLimitTransitionRegionWidthUnits=deg  UpperLimitSpecify=on  UpperLimitBound=0.802851455917  UpperLimitBoundUnits=rad  UpperLimitStiffness=1e4  UpperLimitStiffnessUnits=N*m/deg  UpperLimitDamping=10  UpperLimitDampingUnits=N*m/(deg/s)  UpperLimitTransitionRegionWidth=0.1  UpperLimitTransitionRegionWidthUnits=deg  PositionTargetSpecify=on  PositionTargetPriority=High  PositionTargetValue=0  PositionTargetValueUnits=rad  VelocityTargetSpecify=on  VelocityTargetPriority=High  VelocityTargetValue=0  VelocityTargetValueUnits=deg/s
  FL_thigh : Subsystem
  FL_thigh_joint : sm_lib/Joints/Revolute Joint  JointMode=Normal  SenseConstraintForce=off  SenseConstraintForceX=off  SenseConstraintForceY=off  SenseConstraintForceZ=off  SenseConstraintTorque=off  SenseConstraintTorqueX=off  SenseConstraintTorqueY=off  SenseConstraintTorqueZ=off  SenseTotalForce=off  SenseTotalForceX=off  SenseTotalForceY=off  SenseTotalForceZ=off  SenseTotalTorque=off  SenseTotalTorqueX=off  SenseTotalTorqueY=off  SenseTotalTorqueZ=off  CompositeWrenchDir=FollowerOnBase  CompositeWrenchFrame=BaseFrame  EquilibriumPosition=0  EquilibriumPositionUnits=deg  SpringStiffness=0  SpringStiffnessUnits=N*m/deg  DampingCoefficient=0.01  DampingCoefficientUnits=kg*m^2/(rad*s)  TorqueActuationMode=InputTorque  MotionActuationMode=ComputedMotion  SensePosition=on  SenseVelocity=on  SenseAcceleration=off  SenseTorqueForce=on  SenseLowerLimitTorqueForce=off  SenseUpperLimitTorqueForce=off  LowerLimitSpecify=on  LowerLimitBound=-1.0471975512  LowerLimitBoundUnits=rad  LowerLimitStiffness=1e4  LowerLimitStiffnessUnits=N*m/deg  LowerLimitDamping=10  LowerLimitDampingUnits=N*m/(deg/s)  LowerLimitTransitionRegionWidth=0.1  LowerLimitTransitionRegionWidthUnits=deg  UpperLimitSpecify=on  UpperLimitBound=4.18879020479  UpperLimitBoundUnits=rad  UpperLimitStiffness=1e4  UpperLimitStiffnessUnits=N*m/deg  UpperLimitDamping=10  UpperLimitDampingUnits=N*m/(deg/s)  UpperLimitTransitionRegionWidth=0.1  UpperLimitTransitionRegionWidthUnits=deg  PositionTargetSpecify=on  PositionTargetPriority=High  PositionTargetValue=1  PositionTargetValueUnits=rad  VelocityTargetSpecify=on  VelocityTargetPriority=High  VelocityTargetValue=0  VelocityTargetValueUnits=deg/s
  FL_thigh_shoulder : Subsystem
  Leg Logger : Subsystem
  Leg Logger7 : Subsystem
  Leg Logger8 : Subsystem
  Mux : Mux  Inputs=3
  Mux1 : Mux  Inputs=3
  PS-Simulink Converter{1..12} (12 alike) : nesl_utility/PS-Simulink Converter  PhysicalDomain=network_engine_domain  SubClassName=ps_output  LeftPortType=input  RightPortType=output  PseudoPeriodic=off  Frequencies=[]  VectorFormat=inherit  Unit=inherit  AffineConversion=off
  Separate Torques : MATLAB Function  TreatAsAtomicUnit=on
  Simulink-PS Converter : nesl_utility/Simulink-PS Converter  PhysicalDomain=network_engine_domain  SubClassName=ps_input  LeftPortType=input  RightPortType=output  PseudoPeriodic=off  Frequencies=[]  NoiseDistribution=none  NoiseParameters=[]  Unit=1  AffineConversion=off  FilteringAndDerivatives=provide  SimscapeFilterOrder=1  InputFilterTimeConstant=0.001  UdotUserProvided=0
  Simulink-PS Converter1 : nesl_utility/Simulink-PS Converter  PhysicalDomain=network_engine_domain  SubClassName=ps_input  LeftPortType=input  RightPortType=output  PseudoPeriodic=off  Frequencies=[]  NoiseDistribution=none  NoiseParameters=[]  Unit=1  AffineConversion=off  FilteringAndDerivatives=provide  SimscapeFilterOrder=1  InputFilterTimeConstant=0.001  UdotUserProvided=0
  Simulink-PS Converter2 : nesl_utility/Simulink-PS Converter  PhysicalDomain=network_engine_domain  SubClassName=ps_input  LeftPortType=input  RightPortType=output  PseudoPeriodic=off  Frequencies=[]  NoiseDistribution=none  NoiseParameters=[]  Unit=1  AffineConversion=off  FilteringAndDerivatives=provide  SimscapeFilterOrder=1  InputFilterTimeConstant=0.001  UdotUserProvided=0
  Transform Sensor : sm_lib/Frames and Transforms/Transform Sensor  MeasurementFrame=World  SenseAngle=off  SenseAxis=off  SenseQ=off  SenseR=off  SenseRotationSequence=off  RotationSequence=XYX  SenseOmegaX=off  SenseOmegaY=off  SenseOmegaZ=off  SenseQDot=off  SenseRDot=off  SenseAlphaX=off  SenseAlphaY=off  SenseAlphaZ=off  SenseQDDot=off  SenseRDDot=off  SenseX=on  SenseY=on  SenseZ=on  SenseRad=off  SenseAzim=off  SenseDist=off  SenseInc=off  SenseXDot=on  SenseYDot=on  SenseZDot=on  SenseRadDot=off  SenseAzimDot=off  SenseDistDot=off  SenseIncDot=off  SenseXDDot=off  SenseYDDot=off  SenseZDDot=off  SenseRadDDot=off  SenseAzimDDot=off  SenseDistDDot=off  SenseIncDDot=off
  Velocity Concat : Concatenate  NumInputs=3
  Leg Connection : PMIOPort  Side=Left
  Thigh Contact : PMIOPort  Port=2  Side=Left
  Foot Contact : PMIOPort  Port=3  Side=Left
  World Frame : PMIOPort  Port=4  Side=Left
  Angle Vector : Outport
  Velocity Vector : Outport  Port=2
  " Foot Pos" : Outport  Port=3
  " Foot Vel" : Outport  Port=4
  wires:
  torque_vector/1 -> Separate Torques/1(torque_vector)
  Separate Torques/2(thigh_torque) -> Simulink-PS Converter1/1
  Separate Torques/1(hip_torque) -> Simulink-PS Converter/1
  Separate Torques/3(calf_torque) -> Simulink-PS Converter2/1
  PS-Simulink Converter4/1 -> Velocity Concat/1
  PS-Simulink Converter3/1 -> Angle Concat/3
  PS-Simulink Converter1/1 -> Angle Concat/1
  PS-Simulink Converter6/1 -> Velocity Concat/3
  PS-Simulink Converter5/1 -> Velocity Concat/2
  PS-Simulink Converter2/1 -> Angle Concat/2
  Velocity Concat/1 -> Velocity Vector/1
  Angle Concat/1 -> Angle Vector/1
  PS-Simulink Converter11/1 -> Mux1/2
  PS-Simulink Converter8/1 -> Mux/2
  PS-Simulink Converter9/1 -> Mux/3
  PS-Simulink Converter7/1 -> Mux/1
  Mux/1 -> " Foot Pos"/1
  Mux1/1 -> " Foot Vel"/1
  PS-Simulink Converter10/1 -> Mux1/1
  PS-Simulink Converter12/1 -> Mux1/3
  connections:
  FL_hip/RConn1 -- FL_thigh_joint/LConn1
  FL_calf/LConn1 -- FL_calf_joint/RConn1
  FL_hip/RConn2 -- FL_hip_fixed/LConn1
  FL_hip_fixed/RConn1 -- FL_thigh_shoulder/LConn1
  FL_thigh/RConn2 -- Thigh Contact/RConn1
  FL_calf_joint/LConn1 -- FL_thigh/RConn1
  Leg Logger8/LConn3 -- FL_hip_joint/RConn4
  FL_calf/RConn1 -- FL_foot_fixed/LConn1
  FL_calf_joint/RConn4 -- Leg Logger/LConn3
  Leg Logger7/LConn2 -- PS-Simulink Converter5/LConn1 -- FL_thigh_joint/RConn3
  FL_thigh/LConn1 -- FL_thigh_joint/RConn1
  FL_calf_joint/RConn2 -- PS-Simulink Converter3/LConn1 -- Leg Logger/LConn1
  Leg Logger8/LConn2 -- PS-Simulink Converter4/LConn1 -- FL_hip_joint/RConn3
  FL_hip_joint/LConn1 -- Leg Connection/RConn1
  FL_calf_joint/RConn3 -- PS-Simulink Converter6/LConn1 -- Leg Logger/LConn2
  FL_hip/LConn1 -- FL_hip_joint/RConn1
  Leg Logger7/LConn3 -- FL_thigh_joint/RConn4
  Leg Logger8/LConn1 -- PS-Simulink Converter1/LConn1 -- FL_hip_joint/RConn2
  Leg Logger7/LConn1 -- FL_thigh_joint/RConn2 -- PS-Simulink Converter2/LConn1
  FL_foot/LConn1 -- Transform Sensor/RConn1 -- FL_foot_fixed/RConn1
  FL_foot/LConn2 -- Foot Contact/RConn1
  Simulink-PS Converter1/RConn1 -- FL_thigh_joint/LConn2
  Simulink-PS Converter/RConn1 -- FL_hip_joint/LConn2
  Simulink-PS Converter2/RConn1 -- FL_calf_joint/LConn2
  Transform Sensor/RConn3 -- PS-Simulink Converter8/LConn1
  Transform Sensor/RConn4 -- PS-Simulink Converter9/LConn1
  World Frame/RConn1 -- Transform Sensor/LConn1
  Transform Sensor/RConn7 -- PS-Simulink Converter12/LConn1
  Transform Sensor/RConn6 -- PS-Simulink Converter11/LConn1
  Transform Sensor/RConn5 -- PS-Simulink Converter10/LConn1
  Transform Sensor/RConn2 -- PS-Simulink Converter7/LConn1
